simulink model "Program_2_Italy_SEIRD_R2018a 2"  (R2018a)
settings: Solver=FixedStepAuto  StartTime=0.0  StopTime=71  FixedStep=0.001  RelTol=1e-9  AbsTol=1e-9
undefined symbols (not defined in the file): beta, D0, E0, gamma1, gamma2, gamma3, I0, L0, N, R0, sigbuilder_block, st1, st2, zeta1, zeta2, zeta3
settings Model: OrderedModelArguments=off  Creator=ismae  LastModifiedBy=ismae
settings SolverCC: SolverResetMethod=Robust
settings DataIOCC: ReturnWorkspaceOutputs=on
settings SFSimCC: SimUseLocalCustomCode=on
settings RTWCC: RTWUseLocalCustomCode=on

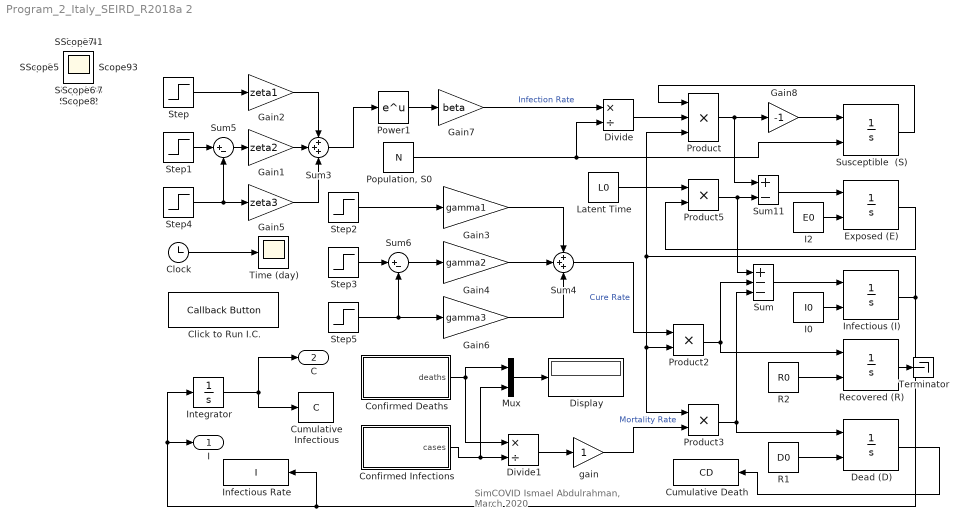
== system Program_2_Italy_SEIRD_R2018a 2 ==
  note: SimCOVID
      | Ismael Abdulrahman, March 2020
  Click to Run I.C. : CallbackButton  Description=Run this callback button first to evaluate the initial values for the parameters  WebBlockId=184
      settings: ClickFcn=|
      | N   = 60*10^6; % Population, Susceptible, N, S0
      | S0  = N;      % Initial value for "Susceptible"
      | I0  = 1;      % Initial value for "Infectious"
      | R0  = 0;      % Initial value for "Removed"
      | E0  = 1;      % Initial value for "Exposed"
      | D0  = 1;      % Initial value for "Death"
      | L0  = 2;      % Latent time
      | st1 = 40;     % starting time 1 (step time)
      | st2 = 52;     % starting time 2 (step time)
      | %==========================================================================
      | %%%%% These are the final values from the optimization obtained by Simulink
      | beta   = 1.971574662033975;
      | gamma1 = 0.019992964106553;
      | gamma2 = 0.015981365215522;
      | gamma3 = 0.564739764641216;
      | zeta1  = -2.179313856128234;
      | zeta2  = -2.080060703203781;
      | zeta3  = -1.046051249951776;
      | I = xlsread('Italy','Italy2','B:B');
      | C = xlsread('Italy','Italy2','D:D');
      | % Note: to calculate the D/I ratio in Simulink, I-variable must be a nonzero variable. Therefore, some
      | % initial days with zero infectious are changed wto one
      | t  = 1:length(C);
      | xy = [t' C];
      | xy0 = [t' I];
  Clock : Clock
  Confirmed Deaths : Subsystem  Tag=STV Subsys  LoadFcn=sigbuilder_block('load');  StartFcn=sigbuilder_block('start');  StopFcn=sigbuilder_block('stop');  ClipboardFcn=sigbuilder_block('clipboard');  mask(Sigbuilder block){tuvar=[0:10]}
      mask help: Simulink:masks:SigbuilderBlock_MD
      mask init:
      | if ~strcmp(get_param(bdroot(gcbh),'SimulationStatus'),'stopped') tuvar = sigbuilder_block('maskInit'); end
      settings: CopyFcn=sigbuilder_block('copy');  DeleteFcn=sigbuilder_block('delete');  ModelCloseFcn=sigbuilder_block('modelClose');  PreSaveFcn=sigbuilder_block('preSave');  PauseFcn=sigbuilder_block('pause');  ContinueFcn=sigbuilder_block('continue');  NameChangeFcn=sigbuilder_block('namechange');  OpenFcn=sigbuilder_block('open',[439.2 183.6 550.8 400.2 ]);  CloseFcn=sigbuilder_block('close');
      mask Display: plot(0, 0, 100, 100,[2, 2, 32, 32, 2], [68, 8, 8, 68, 68],[32, 2], [38, 38], [32, 19, 2],[53, 60, 44], [32, 17, 17, 2],[16, 16, 31, 31]);txt = getActiveGroup(gcbh);text(2, 100, txt,'verticalAlignment', 'top');
  Confirmed Infections : Subsystem  Tag=STV Subsys  LoadFcn=sigbuilder_block('load');  StartFcn=sigbuilder_block('start');  StopFcn=sigbuilder_block('stop');  ClipboardFcn=sigbuilder_block('clipboard');  mask(Sigbuilder block){tuvar=[0:10]}
      mask help: Simulink:masks:SigbuilderBlock_MD
      mask init:
      | if ~strcmp(get_param(bdroot(gcbh),'SimulationStatus'),'stopped') tuvar = sigbuilder_block('maskInit'); end
      settings: CopyFcn=sigbuilder_block('copy');  DeleteFcn=sigbuilder_block('delete');  ModelCloseFcn=sigbuilder_block('modelClose');  PreSaveFcn=sigbuilder_block('preSave');  PauseFcn=sigbuilder_block('pause');  ContinueFcn=sigbuilder_block('continue');  NameChangeFcn=sigbuilder_block('namechange');  OpenFcn=sigbuilder_block('open',[437.6 199.2 550.4 400 ]);  CloseFcn=sigbuilder_block('close');
      mask Display: plot(0, 0, 100, 100,[2, 2, 32, 32, 2], [68, 8, 8, 68, 68],[32, 2], [38, 38], [32, 19, 2],[53, 60, 44], [32, 17, 17, 2],[16, 16, 31, 31]);txt = getActiveGroup(gcbh);text(2, 100, txt,'verticalAlignment', 'top');
  Cumulative Infectious : ToWorkspace  VariableName=C  SaveFormat=Timeseries  SampleTime=-1
  Cumulative Death : ToWorkspace  VariableName=CD  SaveFormat=Timeseries  SampleTime=-1
  Dead (D) : Integrator  InitialConditionSource=external  InitialCondition=10000
  Display : Display
  Divide : Product  Inputs=*/
  Divide1 : Product  Inputs=*/
  Exposed (E) : Integrator  InitialConditionSource=external
  Gain1 : Gain  Gain=zeta2
  Gain2 : Gain  Gain=zeta1
  Gain3 : Gain  Gain=gamma1
  Gain4 : Gain  Gain=gamma2
  Gain5 : Gain  Gain=zeta3
  Gain6 : Gain  Gain=gamma3
  Gain7 : Gain  Gain=beta
  Gain8 : Gain  Gain=-1
  I0 : Constant  Value=I0
  I2 : Constant  Value=E0
  Infectious (I) : Integrator  InitialConditionSource=external
  Infectious Rate : ToWorkspace  VariableName=I  SaveFormat=Timeseries  SampleTime=-1
  Integrator : Integrator
  Latent Time : Constant  Value=L0
  Mux : Mux  Inputs=2
  "Population, S0" : Constant  Value=N
  Power1 : Math  SaturateOnIntegerOverflow=on
  Product : Product  Inputs=3
  Product2 : Product
  Product3 : Product
  Product5 : Product
  R1 : Constant  Value=D0
  R2 : Constant  Value=R0
  Recovered (R) : Integrator  InitialConditionSource=external  InitialCondition=10000
  Step : Step  Time=st1  Before=1  After=0  SampleTime=0
  Step1 : Step  Time=st1  SampleTime=0
  Step2 : Step  Time=st1  Before=1  After=0  SampleTime=0
  Step3 : Step  Time=st1  SampleTime=0
  Step4 : Step  Time=st2  SampleTime=0
  Step5 : Step  Time=st2  SampleTime=0
  Sum : Sum  Inputs=+--
  Sum11 : Sum  Inputs=+-
  Sum3 : Sum  Inputs=+++
  Sum4 : Sum  Inputs=+++
  Sum5 : Sum  Inputs=|+-
  Sum6 : Sum  Inputs=|+-
  Susceptible  (S) : Integrator  InitialConditionSource=external  InitialCondition=10000
  Terminator : Terminator
  Time (day) : Scope
  gain : Gain
  I : Outport
  C : Outport  Port=2
  Scope{,1..43} (44 alike) : Scope
  wires:
  Sum3/1 -> Power1/1
  Product/1 -> Gain8/1, Sum11/1
  Divide/1 -> Product/2
  Sum/1 -> Infectious (I)/1
  I0/1 -> Infectious (I)/2
  "Population, S0"/1 -> Divide/2, Susceptible  (S)/2
  Power1/1 -> Gain7/1
  Step1/1 -> Sum5/1
  Step/1 -> Gain2/1
  Sum5/1 -> Gain1/1
  Gain5/1 -> Sum3/3
  Step4/1 -> Gain5/1, Sum5/2
  Step2/1 -> Gain3/1
  Step3/1 -> Sum6/1
  Step5/1 -> Gain6/1, Sum6/2
  Sum6/1 -> Gain4/1
  Gain1/1 -> Sum3/2
  Gain2/1 -> Sum3/1
  Gain3/1 -> Sum4/1
  Gain4/1 -> Sum4/2
  Gain6/1 -> Sum4/3
  Susceptible  (S)/1 -> Product/1
  Clock/1 -> Time (day)/1
  Product5/1 -> Sum/1, Sum11/2
  I2/1 -> Exposed (E)/2
  Sum11/1 -> Exposed (E)/1
  Exposed (E)/1 -> Product5/2
  R2/1 -> Recovered (R)/2
  R1/1 -> Dead (D)/2
  Latent Time/1 -> Product5/1
  Gain7/1 -> Divide/1  "Infection Rate"
  Sum4/1 -> Product2/1  "Cure Rate"
  Gain8/1 -> Susceptible  (S)/1
  Product2/1 -> Recovered (R)/1, Sum/2
  Product3/1 -> Dead (D)/1, Sum/3
  Confirmed Deaths/1(deaths) -> Mux/1, Divide1/1
  Divide1/1 -> gain/1
  gain/1 -> Product3/2  "Mortality Rate"
  Confirmed Infections/1(cases) -> Mux/2, Divide1/2
  Mux/1 -> Display/1
  Infectious (I)/1 -> Integrator/1, I/1, Infectious Rate/1, Product3/1, Product2/2, Product/3
  Integrator/1 -> Cumulative Infectious/1, C/1
  Dead (D)/1 -> Cumulative Death/1
  Recovered (R)/1 -> Terminator/1

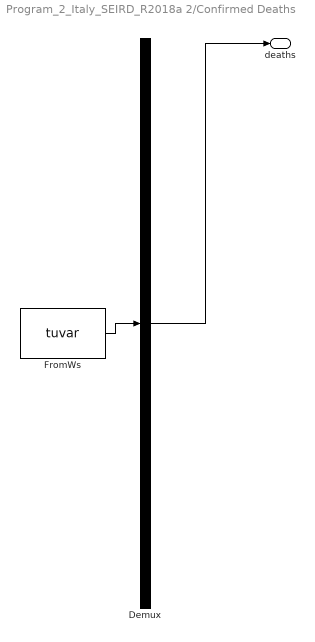
== system Program_2_Italy_SEIRD_R2018a 2/Confirmed Deaths ==
  Demux : Demux  Tag=STV Demux  Outputs=1
  FromWs : FromWorkspace  Tag=STV FromWs  VariableName=tuvar  SampleTime=0
      SigBuilderData=|
      | common.afterFinalStr = 'Extrapolate'
      | common.sampleTime = 0
      | dataSet.timeRange = [1 70]
      | dataSet.name = 'Italy2'
      | sbobj.Groups.Name = 'Italy2'
      | sbobj.Groups.Signals.Name = 'deaths'
      | sbobj.Groups.Signals.XData = [1 2 3 4 5 6 7 8 9 10 11 12 13 14 15 16 17 18 19 20 21 22 23 24 25 26 27 28 29 30 31 32 33 34 35 36 37 38 39 40 41 42 43 44 45 46 47 48 49 50 51 52 53 54 55 56 57 58 59 60 61 62 63 64 65 66 67 68 69 70]
      | sbobj.Groups.Signals.YData = [0 0 0 0 0 0 0 0 0 0 0 0 0 0 0 0 0 0 0 0 0 0 0 2 0 4 5 1 5 4 8 6 17 28 27 41 49 36 133 98 167 196 189 252 173 370 347 347 473 429 625 795 649 601 743 685 660 971 887 758 810 839 727 760 764 681 527 636 604 540]
      | sbobj.Groups.TimeRange = [1 68]
  deaths : Outport  Tag=STV Outport
  wires:
  Demux/1 -> deaths/1
  FromWs/1 -> Demux/1

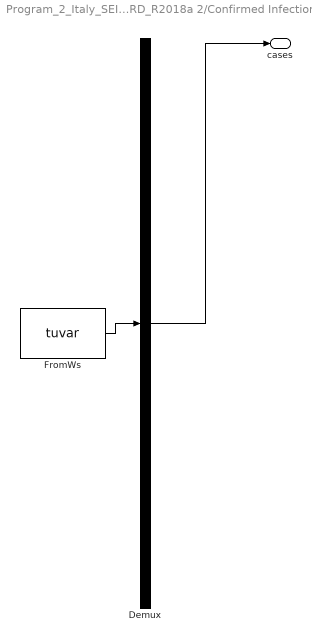
== system Program_2_Italy_SEIRD_R2018a 2/Confirmed Infections ==
  Demux : Demux  Tag=STV Demux  Outputs=1
  FromWs : FromWorkspace  Tag=STV FromWs  VariableName=tuvar  SampleTime=0
      SigBuilderData=|
      | common.afterFinalStr = 'Extrapolate'
      | common.sampleTime = 0
      | dataSet.timeRange = [1 70]
      | dataSet.name = 'Italy2'
      | sbobj.Groups.Name = 'Italy2'
      | sbobj.Groups.Signals.Name = 'cases'
      | sbobj.Groups.Signals.XData = [1 2 3 4 5 6 7 8 9 10 11 12 13 14 15 16 17 18 19 20 21 22 23 24 25 26 27 28 29 30 31 32 33 34 35 36 37 38 39 40 41 42 43 44 45 46 47 48 49 50 51 52 53 54 55 56 57 58 59 60 61 62 63 64 65 66 67 68 69 70]
      | sbobj.Groups.Signals.YData = [3 1 1 1 1 1 1 1 1 1 1 1 1 1 1 1 1 1 1 1 1 1 14 62 53 97 93 78 250 238 240 561 347 466 587 769 778 1247 1492 1797 977 2313 2651 2547 3497 2823 4000 3526 4207 5322 5986 6557 5560 4789 5249 5210 6153 5959 5974 5217 4050 4053 4782 4668 4585 4805 4316 3599 3039 3836]
      | sbobj.Groups.TimeRange = [1 68]
  cases : Outport  Tag=STV Outport
  wires:
  Demux/1 -> cases/1
  FromWs/1 -> Demux/1
